simulink model "Obs_Avoi_with_sta_lin"  (R2023a)
settings: Solver=ode1  StartTime=0  StopTime=30  FixedStep=0.01  RelTol=1e-3
PostLoadFcn:
  | p=1:640; % pixels from left to right
  | 
  | Obtained_angles=(320-p).*(57/640)*pi./180;  % Kinect's horizontal FOV = 57 degrees
  | 
  | S=400; % S = Size of the 2D Map matrix... the highet S is the higher resolution we would end up with - %00 might be high for Embedded computing
values from neighbouring files (symbols this model uses):
  E = 0.3    [Main_Obst_Avoi_sta_lin.m]
  parameters = [R D omega Ts db  E b]    [Main_Obst_Avoi_sta_lin.m]
  Q0 = Qbd    [Main_Obst_Avoi_sta_lin.m]
  R = 0.035    [Main_Obst_Avoi_sta_lin.m]
  T = [R/2 R/2 ... (first row only)    [Main_Obst_Avoi_sta_lin.m]
  thetap = path.States(:,3)    [Main_Obst_Avoi_sta_lin.m]
  x = out.x.Data    [plots.m]
  X0 = p0    [Main_Obst_Avoi_sta_lin.m]
  xp = path.States(:,1)    [Main_Obst_Avoi_sta_lin.m]
  yp = path.States(:,2)    [Main_Obst_Avoi_sta_lin.m]
undefined symbols (not defined in the file or in its folder): gcbh, HIL, JPEG, qc_get_step_size, Video3D, video_display_show
libraries: quarc_library x29, simulink x3
(part 1 of 2)
settings Model: ExtModeTrigDuration=2  Creator=drmadill  LastModifiedBy=Ferna
settings SolverCC: AlgebraicLoopSolver=TrustRegion
settings DebuggingCC: UnderspecifiedInitializationDetection=Classic  MergeDetectMultiDrivingBlocksExec=none  UnconnectedInputMsg=warning  UnconnectedOutputMsg=warning  UnconnectedLineMsg=warning
settings ModelReferenceCC: EnableRefExpFcnMdlSchedulingChecks=on  PropagateSignalLabelsOutOfModel=off

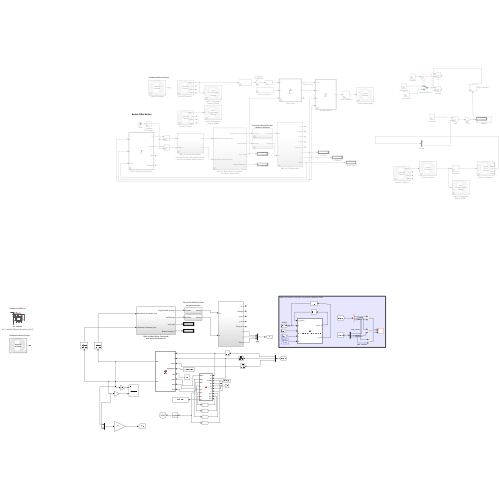
[thumbnail: Simulink's stored preview of the top-level diagram]
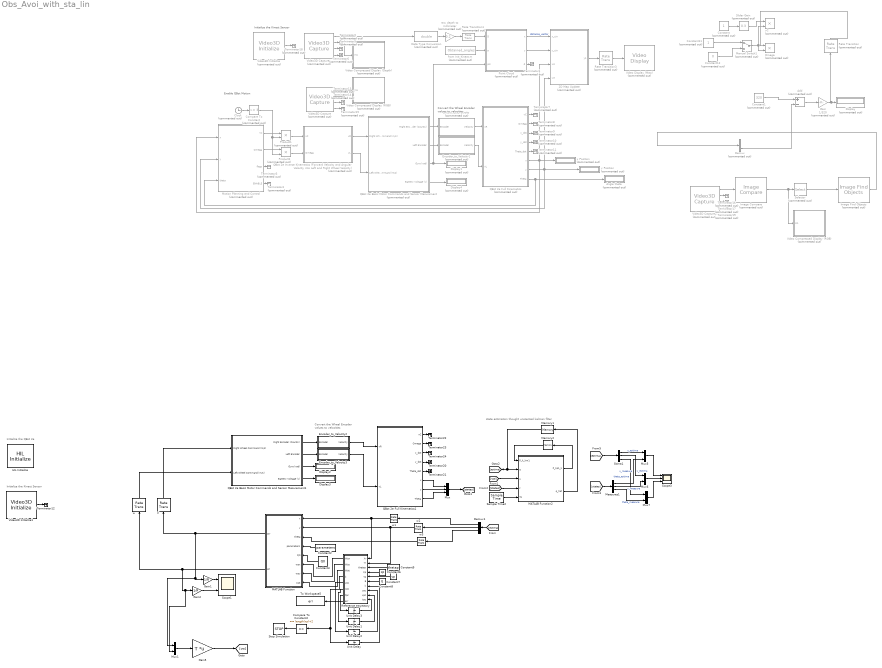
== system Obs_Avoi_with_sta_lin ==
  note: Enable QBot Motion
  note: Initialize the Kinect Sensor
  note: Initialize the QBot 2e
  note: Convert the Wheel Encoder
      | values to velocities
  note: Initialize the Kinect Sensor
  note: Convert the Wheel Encoder
      | values to velocities
  note: state estimation thought unscented kalman filter
  2D Map Update : MATLAB Function  Commented=on  TreatAsAtomicUnit=on  SystemSampleTime=qc_get_step_size
  Add : Sum  Commented=on  Inputs=+-
  Angle theta : Display  Commented=on
  Clock : Clock  Commented=on
  Compare To Constant : simulink/Logic and Bit Operations/Compare To Constant  Commented=on  relop=>=  const=3  OutDataTypeStr=boolean
  Compare To Constant2 : simulink/Logic and Bit Operations/Compare To Constant  relop===  const=length(xp)+2  OutDataTypeStr=boolean
  Constant : Constant  Commented=on
  Constant1 : Constant  Commented=on  Value=320
  Constant11 : Constant  Commented=on
  Constant12 : Constant  Commented=on  Value=0
  Constant2 : Constant  Value=parameters
  Constant3 : Constant  Value=Q0
  Constant6 : Constant  Value=xp
  Constant7 : Constant  Value=yp
  Constant8 : Constant  Value=E
  Constant9 : Constant  Value=thetap
  Data Type Conversion : DataTypeConversion  Commented=on  OutDataTypeStr=double  SaturateOnIntegerOverflow=off  RndMeth=Floor
  Demux : Demux  Commented=on  Outputs=2
  Demux1 : Demux  Outputs=3
  Display : Display  Commented=on
  Display1 : Display  Commented=on
  Display2 : Display
  Display3 : Display
  Display4 : Display  Commented=on
  Encoder_to_Velocity : Subsystem  Commented=on
  Encoder_to_Velocity1 : Subsystem  Commented=on
  Encoder_to_Velocity2 : Subsystem
  Encoder_to_Velocity3 : Subsystem
  Gain : Gain  Commented=on  Gain=1/320
  Gain1 : Gain  Gain=1/R
  Gain2 : Gain  Gain=1/R
  Gain5 : Gain  Gain=T  Multiplication=Matrix(K*u)
  HIL Initialize : quarc_library/Data Acquisition/Generic/Configuration/HIL Initialize  Priority=-99  object_name=HIL-1  board_type=qbot2e  board_number=0@tcpip://localhost:18910  board_options=pwm0_en=1;pwm0_pin=12;pwm1_en=1;pwm1_pin=13;  exclusive=off  active=on  hardware_clocks=[]  clock_modes=[]  initial_clock_frequencies=[]  set_clock_params_at_start=off  set_clock_params_at_switch_in=off  set_clock_frequencies_at_start=off  set_clock_frequencies_at_switch_in=off  analog_input_channels=[0:5]  analog_input_configurations=[]  analog_input_maximums=[16.5 3.3 3.3 3.3 3.3 3.3]  analog_input_minimums=[0 0 0 0 0 0]  set_analog_input_params_at_start=off  set_analog_input_params_at_switch_in=off  analog_output_channels=[]  analog_output_maximums=[]  analog_output_minimums=[]  initial_analog_outputs=[]  final_analog_outputs=[]  watchdog_analog_outputs=[]  set_analog_output_params_at_start=off  set_analog_output_params_at_switch_in=off  set_analog_outputs_at_start=off  set_analog_outputs_at_switch_in=off  set_analog_outputs_at_terminate=off  set_analog_outputs_at_switch_out=off  set_analog_outputs_on_watchdog=off  digital_input_channels=[28:58]  digital_output_channels=[28:31]  digital_output_configuration=[]  initial_digital_outputs=[0]  final_digital_outputs=[0]  watchdog_digital_outputs=[]  set_digital_output_params_at_start=off  set_digital_output_params_at_switch_in=off  set_digital_outputs_at_start=on  set_digital_outputs_at_switch_in=off  set_digital_outputs_at_terminate=on  set_digital_outputs_at_switch_out=off  set_digital_outputs_on_watchdog=off  encoder_channels=[0:1]  quadrature=[4]  encoder_filter_frequency=[]  initial_encoder_counts=[0]  set_encoder_params_at_start=on  set_encoder_params_at_switch_in=off  set_encoder_counts_at_start=on  set_encoder_counts_at_switch_in=off  pwm_channels=[0:1]  pwm_modes=0  pwm_frequency=100e6 / 4095  pwm_configuration=[0]  pwm_alignment=[0]  pwm_polarity=[1]  pwm_leading_deadband=[]  pwm_trailing_deadband=[]  initial_pwm_outputs=[0]  final_pwm_outputs=[0]  watchdog_pwm_outputs=[]  set_pwm_params_at_start=on  set_pwm_params_at_switch_in=off  set_pwm_outputs_at_start=on  set_pwm_outputs_at_switch_in=off  set_pwm_outputs_at_terminate=on  set_pwm_outputs_at_switch_out=off  set_pwm_outputs_on_watchdog=off  other_output_channels=[2000:2001 14000 16000]  initial_other_outputs=[0 0 0 7]  final_other_outputs=[0 0 0 7]  watchdog_other_outputs=[]  set_other_outputs_at_start=on  set_other_outputs_at_switch_in=off  set_other_outputs_at_terminate=on  set_other_outputs_at_switch_out=off  set_other_outputs_on_watchdog=off
  Image Compare : quarc_library/Image Processing/Generic/Image Compare  Commented=on  output_type=Combined (one HxW output)  source=Internal dialog parameters  r_comparison=min <= pixel and pixel <= max  r_minimum=180  r_maximum=255  g_comparison=min <= pixel and pixel <= max  g_minimum=0  g_maximum=50  b_comparison=min <= pixel and pixel <= max  b_minimum=0  b_maximum=50
      settings: SourceProductName=QUARC Targets
  Image Find Objects : quarc_library/Image Processing/Generic/Image Find Objects  Commented=on  num_objects=1  connectivity=8 directions (N, NE, E, SE, S, SW, W, NW)  sort_order=Sort by number of pixels  min_pixels=10  max_pixels=intmax('uint32')  largest=on  exclude_at_edges=off  variable_size=off  use_complex=off
      settings: SourceProductName=QUARC Targets
  MATLAB Function : MATLAB Function  TreatAsAtomicUnit=on
  MATLAB Function2 : MATLAB Function  TreatAsAtomicUnit=on
  Manual Switch1 : ManualSwitch  Commented=on
  Measures1 : Demux  Outputs=3
  Memory1 : Memory  InitialCondition=X0
  Memory2 : Memory  InitialCondition=1e-6*eye(3)
  Motion Planning and Control : MATLAB Function  Commented=on  TreatAsAtomicUnit=on  SystemSampleTime=qc_get_step_size
  Mux : Mux  Inputs=3
  Mux{1,5..7} (4 alike) : Mux  Inputs=2
  Omega : Product  Commented=on  Inputs=**
  Point Cloud : MATLAB Function  Commented=on  TreatAsAtomicUnit=on
  Product1 : Product  Commented=on  RndMeth=Zero
  Product2 : Product  Commented=on  RndMeth=Zero
  QBot 2e Basic Motor Commands and Sensor Mesurement : Subsystem  Commented=on
  QBot 2e Basic Motor Commands and Sensor Mesurement1 : Subsystem
  QBot 2e Full Kinematics : Subsystem  Commented=on
  QBot 2e Full Kinematics1 : Subsystem
  QBot 2e Inverse Kinematics (Forward Velocity and Angular Velocity into Left and Right Wheel Velocity) : Subsystem  Commented=on
  Rate Transition : RateTransition  Commented=on
  Rate Transition1 : RateTransition  Commented=on
  Rate Transition3 : RateTransition  Commented=on
  Reference trayectory : MATLAB Function  TreatAsAtomicUnit=on
  Sample Time2 : quarc_library/Sources/Time/Sample Time  Priority=-99  sample_time=Ts
  Scope1 : Scope  NumInputPorts=2
  Scope3 : Scope  NumInputPorts=3
  Selector : Selector  Commented=on  NumberOfDimensions=2  InputPortWidth=3  IndexOptions=Index vector (dialog),Select all  Indices=[300:480],1  OutputSizes=1,1
  Slider Gain : simulink/Math Operations/Slider Gain  Commented=on  gain=0.3  low=-1  high=1
  Stima1 : Demux  Outputs=3
  Stop Simulation : Stop
  Terminator{1..11,13..19} (18 alike) : Terminator  Commented=on
  Terminator{12,20..24} (6 alike) : Terminator
  To Workspace5 : ToWorkspace  VariableName=err  SaveFormat=Timeseries  SampleTime=-1
  Unit Delay : UnitDelay  InitialCondition=1  SampleTime=0.15  HasFrameUpgradeWarning=on
  Unit Delay1 : UnitDelay  InitialCondition=xp(1)  SampleTime=-1  HasFrameUpgradeWarning=on
  Unit Delay2 : UnitDelay  InitialCondition=yp(1)  SampleTime=-1  HasFrameUpgradeWarning=on
  Unit Delay3 : UnitDelay  InitialCondition=thetap(1)  SampleTime=-1  HasFrameUpgradeWarning=on
  V : RateTransition
  Video Compressed Display (Depth) : Subsystem  Commented=on  LoadFcn=set_param(gcbh, 'UserData', gcb);  StartFcn=video_display_show([gcb, '/Video Display'], 'add', gcb);  mask(Video Compressed Display){algorithm=JPEG, quality=50, sample_time=-1, use_hardware=on}
      mask prompts: algorithm "Compression algorithm:"; quality "Compression quality (0-100):"; sample_time "Sample time (seconds):"; use_hardware "Use hardware acceleration for video display"
      mask help: Displays a video stream on the host, using compression to minimize bandwidth.
      mask init:
      | qc_set_display('Video\nCompressed\nDisplay');
      settings: UndoDeleteFcn=set_param(gcbh, 'UserData', gcb);  OpenFcn=video_display_show([gcb, '/Video Display'], 'show', gcb);  PreDeleteFcn=video_display_show([gcb, '/Video Display'], 'delete');
      settings: CopyFcn=|
      | set_param(gcbh, 'UserData', gcb);
      | set_param(gcbh, 'LinkStatus', 'none');
      settings: NameChangeFcn=|
      | video_display_show([get_param(gcbh, 'UserData'), '/Video Display'], 'rename', [gcb, '/Video Display']);
      | video_display_show([gcb, '/Video Display'], 'add', gcb);
      | set_param(gcbh, 'UserData', gcb);
      mask Help: web(qc_get_block_help_path(gcb));
      mask TypeOptions algorithm: Image Compress/algorithm
      mask TypeOptions quality: Image Compress/quality
      mask TypeOptions sample_time: Video Display/sample_time
      mask TypeOptions use_hardware: Video Display/use_hardware
      mask Display:
      | patch([0.98591 0.98591 0.62618 0.59072 0.56147   0.536   0.536  0.5441 0.56912 0.59207 0.60881 0.62276 0.63527 0.64364  0.6485  0.6485 0.64706 0.64499 0.63662 0.62411 0.61232 0.59837 0.58307 0.56147   0.536   0.536  0.5441  0.5747 0.60953 0.63662 0.67001  0.7034 0.72851 0.75425 0.77927 0.80294 0.82454 0.84119 0.85865 0.87395 0.88574 0.89339  0.8969 0.89969 0.89969 0.89267  0.8816 0.87044 0.85649  0.8384 0.81824 0.80294 0.78764 0.77513 0.76676 0.75776 0.76397 0.77513 0.79178 0.80987 0.82796 0.84326 0.86207 0.98528],[0.18689 0.05522 0.05522 0.05171 0.05171    0.05 0.18338 0.18338 0.19148 0.20435 0.22298 0.24863 0.28589 0.33125 0.38138 0.55139 0.59801 0.63761 0.68189 0.72149 0.74939 0.76694 0.77855 0.79367 0.79952 0.92768 0.92768 0.92768 0.92417 0.92066 0.91364  0.9032 0.89384 0.88106 0.86594 0.85073 0.82634 0.80537 0.77855 0.74363 0.70403 0.65858 0.61079 0.59099 0.41513 0.37202 0.31847 0.29048 0.25556 0.23342  0.2102 0.19382 0.18221 0.17285 0.16943 0.16124  0.1589 0.16241 0.16709 0.17168  0.1787 0.18221 0.18689 0.18689],[0.9,0.90,0.91])
      | patch([0.536 0.52601 0.46823 0.44528 0.41603 0.39101 0.35555 0.33116 0.31451 0.29291  0.2804 0.26717 0.25322 0.23999 0.22406 0.20732 0.19337 0.17528 0.15935 0.14396 0.13217 0.11759 0.10922 0.10085 0.09671 0.09392 0.09041 0.08906 0.08906 0.09464  0.0995 0.10778 0.11894 0.13145 0.14675 0.16349 0.17672 0.19409 0.20732 0.22406 0.23999 0.26159 0.27833 0.29849 0.31793 0.33602 0.35411 0.37085 0.39245 0.41603   0.536   0.536 0.53159 0.46409   0.446 0.42026 0.39587 0.37571 0.36113 0.34925 0.34088 0.33809 0.33809 0.34088 0.34583 0.35627 0.36392 0.38129 0.39587 0.41117 0.42719 0.44672  0.4676 0.48353 0.48353 0.52394   0.536],[0.05 0.04829 0.04712 0.04712 0.04829 0.05063 0.05405 0.05873 0.06107 0.06692 0.07043 0.07619 0.08087 0.08672 0.09482 0.10652 0.11696 0.13325  0.1508 0.17168 0.19499 0.22415 0.25439 0.28472 0.31379 0.35456 0.38489 0.41513 0.58055 0.63878 0.68774 0.72149 0.75641 0.78089 0.80537 0.82859 0.84029 0.85658 0.86594 0.87404  0.8834 0.89267 0.90086 0.90788 0.91247 0.91832 0.92066   0.923 0.92651 0.92768 0.92768 0.79952 0.79952 0.79952 0.79718 0.78899 0.77153 0.75056 0.72149 0.68072 0.62249  0.5549 0.41396 0.37085 0.33242 0.28121 0.25205 0.22181 0.20552 0.19499 0.18572 0.18221 0.17753 0.17636 0.17753  0.1787  0.1787],[0.9,0.90,0.91])
      | disp('Video\nCompressed\nDisplay');
  Video Compressed Display (RGB) : Subsystem  Commented=on  LoadFcn=set_param(gcbh, 'UserData', gcb);  StartFcn=video_display_show([gcb, '/Video Display'], 'add', gcb);  mask(Video Compressed Display){algorithm=JPEG, quality=50, sample_time=-1, use_hardware=on}
      mask prompts: algorithm "Compression algorithm:"; quality "Compression quality (0-100):"; sample_time "Sample time (seconds):"; use_hardware "Use hardware acceleration for video display"
      mask help: Displays a video stream on the host, using compression to minimize bandwidth.
      mask init:
      | qc_set_display('Video\nCompressed\nDisplay');
      settings: UndoDeleteFcn=set_param(gcbh, 'UserData', gcb);  OpenFcn=video_display_show([gcb, '/Video Display'], 'show', gcb);  PreDeleteFcn=video_display_show([gcb, '/Video Display'], 'delete');
      settings: CopyFcn=|
      | set_param(gcbh, 'UserData', gcb);
      | set_param(gcbh, 'LinkStatus', 'none');
      settings: NameChangeFcn=|
      | video_display_show([get_param(gcbh, 'UserData'), '/Video Display'], 'rename', [gcb, '/Video Display']);
      | video_display_show([gcb, '/Video Display'], 'add', gcb);
      | set_param(gcbh, 'UserData', gcb);
      mask Help: web(qc_get_block_help_path(gcb));
      mask TypeOptions algorithm: Image Compress/algorithm
      mask TypeOptions quality: Image Compress/quality
      mask TypeOptions sample_time: Video Display/sample_time
      mask TypeOptions use_hardware: Video Display/use_hardware
      mask Display:
      | patch([0.98591 0.98591 0.62618 0.59072 0.56147   0.536   0.536  0.5441 0.56912 0.59207 0.60881 0.62276 0.63527 0.64364  0.6485  0.6485 0.64706 0.64499 0.63662 0.62411 0.61232 0.59837 0.58307 0.56147   0.536   0.536  0.5441  0.5747 0.60953 0.63662 0.67001  0.7034 0.72851 0.75425 0.77927 0.80294 0.82454 0.84119 0.85865 0.87395 0.88574 0.89339  0.8969 0.89969 0.89969 0.89267  0.8816 0.87044 0.85649  0.8384 0.81824 0.80294 0.78764 0.77513 0.76676 0.75776 0.76397 0.77513 0.79178 0.80987 0.82796 0.84326 0.86207 0.98528],[0.18689 0.05522 0.05522 0.05171 0.05171    0.05 0.18338 0.18338 0.19148 0.20435 0.22298 0.24863 0.28589 0.33125 0.38138 0.55139 0.59801 0.63761 0.68189 0.72149 0.74939 0.76694 0.77855 0.79367 0.79952 0.92768 0.92768 0.92768 0.92417 0.92066 0.91364  0.9032 0.89384 0.88106 0.86594 0.85073 0.82634 0.80537 0.77855 0.74363 0.70403 0.65858 0.61079 0.59099 0.41513 0.37202 0.31847 0.29048 0.25556 0.23342  0.2102 0.19382 0.18221 0.17285 0.16943 0.16124  0.1589 0.16241 0.16709 0.17168  0.1787 0.18221 0.18689 0.18689],[0.9,0.90,0.91])
      | patch([0.536 0.52601 0.46823 0.44528 0.41603 0.39101 0.35555 0.33116 0.31451 0.29291  0.2804 0.26717 0.25322 0.23999 0.22406 0.20732 0.19337 0.17528 0.15935 0.14396 0.13217 0.11759 0.10922 0.10085 0.09671 0.09392 0.09041 0.08906 0.08906 0.09464  0.0995 0.10778 0.11894 0.13145 0.14675 0.16349 0.17672 0.19409 0.20732 0.22406 0.23999 0.26159 0.27833 0.29849 0.31793 0.33602 0.35411 0.37085 0.39245 0.41603   0.536   0.536 0.53159 0.46409   0.446 0.42026 0.39587 0.37571 0.36113 0.34925 0.34088 0.33809 0.33809 0.34088 0.34583 0.35627 0.36392 0.38129 0.39587 0.41117 0.42719 0.44672  0.4676 0.48353 0.48353 0.52394   0.536],[0.05 0.04829 0.04712 0.04712 0.04829 0.05063 0.05405 0.05873 0.06107 0.06692 0.07043 0.07619 0.08087 0.08672 0.09482 0.10652 0.11696 0.13325  0.1508 0.17168 0.19499 0.22415 0.25439 0.28472 0.31379 0.35456 0.38489 0.41513 0.58055 0.63878 0.68774 0.72149 0.75641 0.78089 0.80537 0.82859 0.84029 0.85658 0.86594 0.87404  0.8834 0.89267 0.90086 0.90788 0.91247 0.91832 0.92066   0.923 0.92651 0.92768 0.92768 0.79952 0.79952 0.79952 0.79718 0.78899 0.77153 0.75056 0.72149 0.68072 0.62249  0.5549 0.41396 0.37085 0.33242 0.28121 0.25205 0.22181 0.20552 0.19499 0.18572 0.18221 0.17753 0.17636 0.17753  0.1787  0.1787],[0.9,0.90,0.91])
      | disp('Video\nCompressed\nDisplay');
  "Video Compressed Display (RGB) " : Subsystem  Commented=on  LoadFcn=set_param(gcbh, 'UserData', gcb);  StartFcn=video_display_show([gcb, '/Video Display'], 'add', gcb);  mask(Video Compressed Display){algorithm=JPEG, quality=50, sample_time=-1, use_hardware=on}
      mask prompts: algorithm "Compression algorithm:"; quality "Compression quality (0-100):"; sample_time "Sample time (seconds):"; use_hardware "Use hardware acceleration for video display"
      mask help: Displays a video stream on the host, using compression to minimize bandwidth.
      mask init:
      | qc_set_display('Video\nCompressed\nDisplay');
      settings: UndoDeleteFcn=set_param(gcbh, 'UserData', gcb);  OpenFcn=video_display_show([gcb, '/Video Display'], 'show', gcb);  PreDeleteFcn=video_display_show([gcb, '/Video Display'], 'delete');
      settings: CopyFcn=|
      | set_param(gcbh, 'UserData', gcb);
      | set_param(gcbh, 'LinkStatus', 'none');
      settings: NameChangeFcn=|
      | video_display_show([get_param(gcbh, 'UserData'), '/Video Display'], 'rename', [gcb, '/Video Display']);
      | video_display_show([gcb, '/Video Display'], 'add', gcb);
      | set_param(gcbh, 'UserData', gcb);
      mask Help: web(qc_get_block_help_path(gcb));
      mask TypeOptions algorithm: Image Compress/algorithm
      mask TypeOptions quality: Image Compress/quality
      mask TypeOptions sample_time: Video Display/sample_time
      mask TypeOptions use_hardware: Video Display/use_hardware
      mask Display:
      | patch([0.98591 0.98591 0.62618 0.59072 0.56147   0.536   0.536  0.5441 0.56912 0.59207 0.60881 0.62276 0.63527 0.64364  0.6485  0.6485 0.64706 0.64499 0.63662 0.62411 0.61232 0.59837 0.58307 0.56147   0.536   0.536  0.5441  0.5747 0.60953 0.63662 0.67001  0.7034 0.72851 0.75425 0.77927 0.80294 0.82454 0.84119 0.85865 0.87395 0.88574 0.89339  0.8969 0.89969 0.89969 0.89267  0.8816 0.87044 0.85649  0.8384 0.81824 0.80294 0.78764 0.77513 0.76676 0.75776 0.76397 0.77513 0.79178 0.80987 0.82796 0.84326 0.86207 0.98528],[0.18689 0.05522 0.05522 0.05171 0.05171    0.05 0.18338 0.18338 0.19148 0.20435 0.22298 0.24863 0.28589 0.33125 0.38138 0.55139 0.59801 0.63761 0.68189 0.72149 0.74939 0.76694 0.77855 0.79367 0.79952 0.92768 0.92768 0.92768 0.92417 0.92066 0.91364  0.9032 0.89384 0.88106 0.86594 0.85073 0.82634 0.80537 0.77855 0.74363 0.70403 0.65858 0.61079 0.59099 0.41513 0.37202 0.31847 0.29048 0.25556 0.23342  0.2102 0.19382 0.18221 0.17285 0.16943 0.16124  0.1589 0.16241 0.16709 0.17168  0.1787 0.18221 0.18689 0.18689],[0.9,0.90,0.91])
      | patch([0.536 0.52601 0.46823 0.44528 0.41603 0.39101 0.35555 0.33116 0.31451 0.29291  0.2804 0.26717 0.25322 0.23999 0.22406 0.20732 0.19337 0.17528 0.15935 0.14396 0.13217 0.11759 0.10922 0.10085 0.09671 0.09392 0.09041 0.08906 0.08906 0.09464  0.0995 0.10778 0.11894 0.13145 0.14675 0.16349 0.17672 0.19409 0.20732 0.22406 0.23999 0.26159 0.27833 0.29849 0.31793 0.33602 0.35411 0.37085 0.39245 0.41603   0.536   0.536 0.53159 0.46409   0.446 0.42026 0.39587 0.37571 0.36113 0.34925 0.34088 0.33809 0.33809 0.34088 0.34583 0.35627 0.36392 0.38129 0.39587 0.41117 0.42719 0.44672  0.4676 0.48353 0.48353 0.52394   0.536],[0.05 0.04829 0.04712 0.04712 0.04829 0.05063 0.05405 0.05873 0.06107 0.06692 0.07043 0.07619 0.08087 0.08672 0.09482 0.10652 0.11696 0.13325  0.1508 0.17168 0.19499 0.22415 0.25439 0.28472 0.31379 0.35456 0.38489 0.41513 0.58055 0.63878 0.68774 0.72149 0.75641 0.78089 0.80537 0.82859 0.84029 0.85658 0.86594 0.87404  0.8834 0.89267 0.90086 0.90788 0.91247 0.91832 0.92066   0.923 0.92651 0.92768 0.92768 0.79952 0.79952 0.79952 0.79718 0.78899 0.77153 0.75056 0.72149 0.68072 0.62249  0.5549 0.41396 0.37085 0.33242 0.28121 0.25205 0.22181 0.20552 0.19499 0.18572 0.18221 0.17753 0.17636 0.17753  0.1787  0.1787],[0.9,0.90,0.91])
      | disp('Video\nCompressed\nDisplay');
  Video Display (Map) : quarc_library/Multimedia/Video Display  Tag=Obs_Avoi_with_sta_lin/Video Display (Map)  Commented=on  sample_time=-1  use_hardware=on
  Video3D Capture : quarc_library/Multimedia/Video3D Capture  Commented=on  object_name=Video3D-1  stream_type=RGB  stream_index=0  resolution=640 x 480  width=640  height=480  output_format=MATLAB RGB (HxWx3)  data_type=uint8  sample_time=qc_get_step_size * ceil(0.033 / qc_get_step_size)  camera_intrinsics=off  depth_scale=off  brightness_override=off  brightness=50.0  contrast_override=off  contrast=50.0  hue_override=off  hue=50.0  saturation_override=off  saturation=50.0  sharpness_override=off  sharpness=50.0  gamma_override=off  gamma=50.0  gain_override=off  gain=50.0  backlightcompensation_override=off  backlightcompensation=50.0  whitebalance_override=Automatic white balance  whitebalance=50.0  exposure_override=Automatic exposure  exposure=30.0  emitter=Enable laser emitter  preset=Do not set camera presets
  Video3D Capture1 : quarc_library/Multimedia/Video3D Capture  Commented=on  object_name=Video3D-1  stream_type=Depth  stream_index=0  resolution=640 x 480  width=640  height=480  output_format=MATLAB greyscale (HxW)  data_type=uint16  sample_time=qc_get_step_size * ceil(0.033 / qc_get_step_size)  camera_intrinsics=off  depth_scale=off  brightness_override=off  brightness=50.0  contrast_override=off  contrast=50.0  hue_override=off  hue=50.0  saturation_override=off  saturation=50.0  sharpness_override=off  sharpness=50.0  gamma_override=off  gamma=50.0  gain_override=off  gain=50.0  backlightcompensation_override=off  backlightcompensation=50.0  whitebalance_override=Automatic white balance  whitebalance=50.0  exposure_override=Automatic exposure  exposure=30.0  emitter=Enable laser emitter  preset=Do not set camera presets
  Video3D Capture2 : quarc_library/Multimedia/Video3D Capture  Commented=on  object_name=Video3D-1  stream_type=RGB  stream_index=0  resolution=640 x 480  width=640  height=480  output_format=MATLAB RGB (HxWx3)  data_type=uint8  sample_time=qc_get_step_size * ceil(0.033 / qc_get_step_size)  camera_intrinsics=off  depth_scale=off  brightness_override=off  brightness=50.0  contrast_override=off  contrast=50.0  hue_override=off  hue=50.0  saturation_override=off  saturation=50.0  sharpness_override=off  sharpness=50.0  gamma_override=off  gamma=50.0  gain_override=off  gain=50.0  backlightcompensation_override=off  backlightcompensation=50.0  whitebalance_override=Automatic white balance  whitebalance=50.0  exposure_override=Automatic exposure  exposure=30.0  emitter=Enable laser emitter  preset=Do not set camera presets
  Video3D Initialize : quarc_library/Multimedia/Video3D Initialize  Commented=on  object_name=Video3D-1  source=Device  identifier=0@tcpip://localhost:18911  file=sample.bag  sample_time=qc_get_step_size * ceil(0.033 / qc_get_step_size)  active=on
  Video3D Initialize1 : quarc_library/Multimedia/Video3D Initialize  object_name=Video3D-1  source=Device  identifier=0@tcpip://localhost:18911  file=sample.bag  sample_time=qc_get_step_size * ceil(0.033 / qc_get_step_size)  active=on
  from Init_Kinect.m : Constant  Commented=on  Value=Obtained_angles
  raw depth to millimeter : Gain  Commented=on  Gain=0.2  OutDataTypeStr=single
  vC : Product  Commented=on  Inputs=**
  w : RateTransition
  w1 : RateTransition  OutPortSampleTime=Ts
  w2 : RateTransition  OutPortSampleTime=Ts
  w3 : RateTransition  OutPortSampleTime=Ts
  x Position : Display  Commented=on
  y Position : Display  Commented=on
  wires:
  QBot 2e Basic Motor Commands and Sensor Mesurement/1(Right Encoder (Counts)) -> Encoder_to_Velocity/1(Encoder)
  QBot 2e Full Kinematics/8(Theta) -> Motion Planning and Control/3(theta), Angle theta/1
  QBot 2e Full Kinematics/6(x) -> Motion Planning and Control/1(x), x Position/1, 2D Map Update/3(xin)
  from Init_Kinect.m/1 -> Point Cloud/2(a)
  Point Cloud/1(x) -> 2D Map Update/1(x_cin)  "distance_vector"
  Point Cloud/2(y) -> 2D Map Update/2(y_cin)
  2D Map Update/1(y1) -> Rate Transition3/1
  Video3D Capture1/1 -> Video Compressed Display (Depth)/1(In1), Data Type Conversion/1
  QBot 2e Basic Motor Commands and Sensor Mesurement/3(Gyro (rad)) -> Point Cloud/3(psi), Display1/1
  QBot 2e Basic Motor Commands and Sensor Mesurement/4(Battery Voltage (v)) -> Display4/1
  Encoder_to_Velocity/1(Velocity) -> QBot 2e Full Kinematics/1(vR)
  QBot 2e Inverse Kinematics (Forward Velocity and Angular Velocity into Left and Right Wheel Velocity)/2(vL) -> QBot 2e Basic Motor Commands and Sensor Mesurement/2(Left Wheel Command (m/s))
  QBot 2e Basic Motor Commands and Sensor Mesurement/2(Left Encoder) -> Encoder_to_Velocity1/1(Encoder)
  Encoder_to_Velocity1/1(Velocity) -> QBot 2e Full Kinematics/2(vL)
  Motion Planning and Control/1(Vc) -> Product1/1
  Product1/1 -> QBot 2e Inverse Kinematics (Forward Velocity and Angular Velocity into Left and Right Wheel Velocity)/1(vC)
  Motion Planning and Control/2(Omega) -> Product2/1
  Product2/1 -> QBot 2e Inverse Kinematics (Forward Velocity and Angular Velocity into Left and Right Wheel Velocity)/2(Omega)
  Compare To Constant/1 -> Product2/2, Product1/2
  QBot 2e Inverse Kinematics (Forward Velocity and Angular Velocity into Left and Right Wheel Velocity)/1(vR) -> QBot 2e Basic Motor Commands and Sensor Mesurement/1(Right Wheel Command (m/s))
  Motion Planning and Control/3(flags) -> Terminator3/1
  Motion Planning and Control/4(ENABLE) -> Terminator4/1
  QBot 2e Full Kinematics/7(y) -> y Position/1, 2D Map Update/4(yin), Motion Planning and Control/2(y)
  QBot 2e Full Kinematics/1(vC) -> Terminator7/1
  QBot 2e Full Kinematics/2(Omega) -> Terminator8/1
  QBot 2e Full Kinematics/3(x_dot) -> Terminator9/1
  QBot 2e Full Kinematics/4(y_dot) -> Terminator10/1
  QBot 2e Full Kinematics/5(Theta_dot) -> Terminator11/1
  Rate Transition3/1 -> Video Display (Map)/1
  Video3D Capture/1 -> Video Compressed Display (RGB)/1(In1)
  Point Cloud/3(d) -> Terminator1/1
  Video3D Capture/2 -> Terminator13/1
  Video3D Capture/4 -> Terminator15/1
  Video3D Capture/3 -> Terminator14/1
  Video3D Initialize/1 -> Terminator18/1
  Video3D Capture1/2 -> Terminator2/1
  Video3D Capture1/3 -> Terminator5/1
  Video3D Capture1/4 -> Terminator6/1
  Rate Transition1/1 -> Point Cloud/1(D)
  raw depth to millimeter/1 -> Rate Transition1/1
  Data Type Conversion/1 -> raw depth to millimeter/1
  Clock/1 -> Compare To Constant/1
  Constant/1 -> Slider Gain/1
  Video3D Initialize1/1 -> Terminator12/1
  Video3D Capture2/4 -> Terminator19/1
  Video3D Capture2/2 -> Terminator16/1
  Video3D Capture2/1 -> Image Compare/1
  Video3D Capture2/3 -> Terminator17/1
  Image Compare/1 -> "Video Compressed Display (RGB) "/1(In1), Selector/1
  Selector/1 -> Image Find Objects/1
  Image Find Objects/3 -> Demux/1
  Demux/2 -> Add/2
  Constant1/1 -> Add/1
  Add/1 -> Gain/1
  Gain/1 -> Rate Transition/1, Display/1
  QBot 2e Basic Motor Commands and Sensor Mesurement1/1(Right Encoder (Counts)) -> Encoder_to_Velocity2/1(Encoder)
  QBot 2e Basic Motor Commands and Sensor Mesurement1/2(Left Encoder) -> Encoder_to_Velocity3/1(Encoder)
  QBot 2e Basic Motor Commands and Sensor Mesurement1/4(Battery Voltage (v)) -> Display3/1
  QBot 2e Basic Motor Commands and Sensor Mesurement1/3(Gyro (rad)) -> Display2/1
  QBot 2e Full Kinematics1/4(y_dot) -> Terminator20/1
  QBot 2e Full Kinematics1/3(x_dot) -> Terminator24/1
  Encoder_to_Velocity2/1(Velocity) -> QBot 2e Full Kinematics1/1(vR)
  QBot 2e Full Kinematics1/5(Theta_dot) -> Terminator21/1
  QBot 2e Full Kinematics1/2(Omega) -> Terminator23/1
  QBot 2e Full Kinematics1/1(vC) -> Terminator22/1
  Encoder_to_Velocity3/1(Velocity) -> QBot 2e Full Kinematics1/2(vL)
  QBot 2e Full Kinematics1/6(x) -> Mux/1
  QBot 2e Full Kinematics1/8(Theta) -> Mux/3
  w1/1 -> Reference trayectory/1(Xr), MATLAB Function/1(x)
  w3/1 -> MATLAB Function/3(theta)
  MATLAB Function/1(Wr) -> V/1, Mux1/1, Gain1/1
  Reference trayectory/1(Wpx) -> MATLAB Function/6(wpx)
  Reference trayectory/2(Wpy) -> MATLAB Function/7(wpy)
  Constant2/1 -> MATLAB Function/4(parameters)
  Constant3/1 -> MATLAB Function/5(Q0)
  Slider Gain/1 -> vC/1
  Constant12/1 -> Manual Switch1/2
  Constant11/1 -> Manual Switch1/1
  Manual Switch1/1 -> Omega/2, vC/2
  Rate Transition/1 -> Omega/1
  w2/1 -> Reference trayectory/2(Yr), MATLAB Function/2(y)
  QBot 2e Full Kinematics1/7(y) -> Mux/2
  MATLAB Function/2(Wl) -> w/1, Mux1/2, Gain2/1
  w/1 -> QBot 2e Basic Motor Commands and Sensor Mesurement1/2(Left Wheel Command (m/s))
  V/1 -> QBot 2e Basic Motor Commands and Sensor Mesurement1/1(Right Wheel Command (m/s))
  Gain1/1 -> Scope1/1
  Gain2/1 -> Scope1/2
  Constant6/1 -> Reference trayectory/4(Xp)
  Constant7/1 -> Reference trayectory/5(Yp)
  Constant8/1 -> Reference trayectory/6(E)
  Reference trayectory/4(k) -> Compare To Constant2/1, Unit Delay/1
  Unit Delay/1 -> Reference trayectory/7("k ")
  Unit Delay1/1 -> Reference trayectory/9("xpc ")
  Unit Delay2/1 -> Reference trayectory/8("ypc ")
  Reference trayectory/6(xpc) -> Unit Delay1/1
  Reference trayectory/5(ypc) -> Unit Delay2/1
  Constant9/1 -> Reference trayectory/3(thetap)
  Reference trayectory/7(tpc) -> Unit Delay3/1
  Unit Delay3/1 -> Reference trayectory/10("tpc ")
  Reference trayectory/3(Wpt) -> MATLAB Function/8(wpt)
  Compare To Constant2/1 -> Stop Simulation/1
  Demux1/1 -> w1/1
  Demux1/2 -> w2/1
  Demux1/3 -> w3/1
  Mux1/1 -> Gain5/1
  Reference trayectory/8(err) -> To Workspace5/1
  Stima1/2 -> Mux6/1  "y_estima"
  Measures1/3 -> Mux7/2  "theta_measure"
  Mux7/1 -> Scope3/3
  [states] -> Measures1/1
  Stima1/3 -> Mux7/1  "theta_estima"
  MATLAB Function2/1(P_kp1_k) -> Memory2/1
  Measures1/1 -> Mux5/2  "x_measure"
  Mux6/1 -> Scope3/2
  [estima] -> Stima1/1
  [vw] -> MATLAB Function2/3(u)
  [states] -> MATLAB Function2/4(y)
  Memory2/1 -> MATLAB Function2/1(P_k_km1)
  Sample Time2/1 -> MATLAB Function2/5(Ts)
  MATLAB Function2/2(q_hat) -> Memory1/1
  Stima1/1 -> Mux5/1  "x_estima"
  Mux5/1 -> Scope3/1
  Memory1/1 -> MATLAB Function2/2(q), [estima]
  Measures1/2 -> Mux6/2  "y_measure"
  Mux/1 -> [states]
  [estima] -> Demux1/1
  Gain5/1 -> [vw]

== system Obs_Avoi_with_sta_lin/Encoder_to_Velocity ==
  Encoder : Inport
  Encoder to Distance : Subsystem
  Second-Order Low-Pass Filter2 : quarc_library/Continuous/Second-Order Low-Pass Filter  params_source=Internal (dialog parameters)  input_width=10  input_zeta=1  input_init=0
  Terminator1 : Terminator
  Velocity : Outport  VectorParamsAs1DForOutWhenUnconnected=off
  wires:
  Second-Order Low-Pass Filter2/1 -> Terminator1/1
  Encoder to Distance/1(Wheel Distance (m)) -> Second-Order Low-Pass Filter2/1
  Encoder/1 -> Encoder to Distance/1(Encoder Counts)
  Second-Order Low-Pass Filter2/2 -> Velocity/1

== system Obs_Avoi_with_sta_lin/Encoder_to_Velocity1 ==
  Encoder : Inport
  Encoder to Distance : Subsystem
  Second-Order Low-Pass Filter2 : quarc_library/Continuous/Second-Order Low-Pass Filter  params_source=Internal (dialog parameters)  input_width=10  input_zeta=1  input_init=0
  Terminator1 : Terminator
  Velocity : Outport  VectorParamsAs1DForOutWhenUnconnected=off
  wires:
  Second-Order Low-Pass Filter2/2 -> Velocity/1
  Encoder/1 -> Encoder to Distance/1(Encoder Counts)
  Encoder to Distance/1(Wheel Distance (m)) -> Second-Order Low-Pass Filter2/1
  Second-Order Low-Pass Filter2/1 -> Terminator1/1

== system Obs_Avoi_with_sta_lin/Encoder_to_Velocity2 ==
  Encoder : Inport
  Encoder to Distance : Subsystem
  Second-Order Low-Pass Filter2 : quarc_library/Continuous/Second-Order Low-Pass Filter  params_source=Internal (dialog parameters)  input_width=10  input_zeta=1  input_init=0
  Terminator1 : Terminator
  Velocity : Outport  VectorParamsAs1DForOutWhenUnconnected=off
  wires:
  Second-Order Low-Pass Filter2/1 -> Terminator1/1
  Encoder to Distance/1(Wheel Distance (m)) -> Second-Order Low-Pass Filter2/1
  Encoder/1 -> Encoder to Distance/1(Encoder Counts)
  Second-Order Low-Pass Filter2/2 -> Velocity/1

== system Obs_Avoi_with_sta_lin/Encoder_to_Velocity3 ==
  Encoder : Inport
  Encoder to Distance : Subsystem
  Second-Order Low-Pass Filter2 : quarc_library/Continuous/Second-Order Low-Pass Filter  params_source=Internal (dialog parameters)  input_width=10  input_zeta=1  input_init=0
  Terminator1 : Terminator
  Velocity : Outport  VectorParamsAs1DForOutWhenUnconnected=off
  wires:
  Second-Order Low-Pass Filter2/2 -> Velocity/1
  Encoder/1 -> Encoder to Distance/1(Encoder Counts)
  Encoder to Distance/1(Wheel Distance (m)) -> Second-Order Low-Pass Filter2/1
  Second-Order Low-Pass Filter2/1 -> Terminator1/1

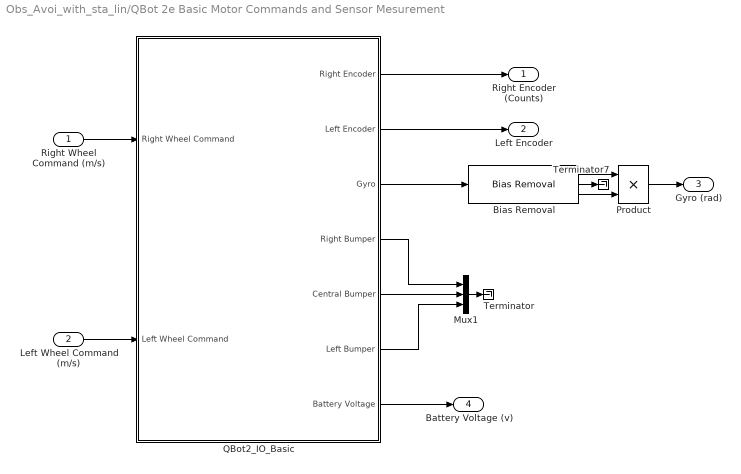
== system Obs_Avoi_with_sta_lin/QBot 2e Basic Motor Commands and Sensor Mesurement ==
  Right Wheel Command (m/s) : Inport
  Left Wheel Command (m/s) : Inport  Port=2
  Bias Removal : quarc_library/Discrete/Bias Removal  start_time=3  end_time=4  switch_id=0  sample_time=qc_get_step_size
      settings: SourceProductName=QUARC Targets
  Mux1 : Mux  Inputs=3
  Product : Product  RndMeth=Zero
  QBot2_IO_Basic : Subsystem
  Terminator : Terminator
  Terminator7 : Terminator
  Right Encoder (Counts) : Outport  VectorParamsAs1DForOutWhenUnconnected=off
  Left Encoder : Outport  Port=2  VectorParamsAs1DForOutWhenUnconnected=off
  Gyro (rad) : Outport  Port=3  VectorParamsAs1DForOutWhenUnconnected=off
  Battery Voltage (v) : Outport  Port=4  VectorParamsAs1DForOutWhenUnconnected=off
  wires:
  QBot2_IO_Basic/4(Right Bumper) -> Mux1/1
  QBot2_IO_Basic/5(Central Bumper) -> Mux1/2
  QBot2_IO_Basic/6(Left Bumper) -> Mux1/3
  Right Wheel Command (m/s)/1 -> QBot2_IO_Basic/1(Right Wheel Command)
  Left Wheel Command (m/s)/1 -> QBot2_IO_Basic/2(Left Wheel Command)
  QBot2_IO_Basic/1(Right Encoder) -> Right Encoder (Counts)/1
  QBot2_IO_Basic/2(Left Encoder) -> Left Encoder/1
  QBot2_IO_Basic/7(Battery Voltage) -> Battery Voltage (v)/1
  Bias Removal/2 -> Terminator7/1
  Bias Removal/1 -> Product/1
  Bias Removal/3 -> Product/2
  Product/1 -> Gyro (rad)/1
  QBot2_IO_Basic/3(Gyro) -> Bias Removal/1
  Mux1/1 -> Terminator/1

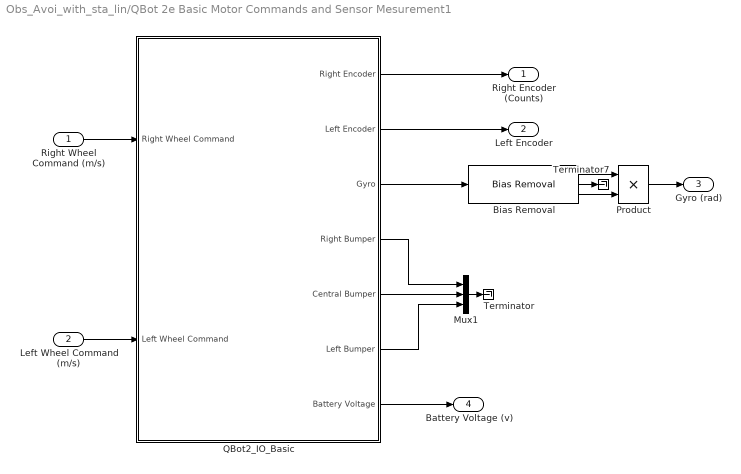
== system Obs_Avoi_with_sta_lin/QBot 2e Basic Motor Commands and Sensor Mesurement1 ==
  Right Wheel Command (m/s) : Inport
  Left Wheel Command (m/s) : Inport  Port=2
  Bias Removal : quarc_library/Discrete/Bias Removal  start_time=3  end_time=4  switch_id=0  sample_time=qc_get_step_size
      settings: SourceProductName=QUARC Targets
  Mux1 : Mux  Inputs=3
  Product : Product  RndMeth=Zero
  QBot2_IO_Basic : Subsystem
  Terminator : Terminator
  Terminator7 : Terminator
  Right Encoder (Counts) : Outport  VectorParamsAs1DForOutWhenUnconnected=off
  Left Encoder : Outport  Port=2  VectorParamsAs1DForOutWhenUnconnected=off
  Gyro (rad) : Outport  Port=3  VectorParamsAs1DForOutWhenUnconnected=off
  Battery Voltage (v) : Outport  Port=4  VectorParamsAs1DForOutWhenUnconnected=off
  wires:
  QBot2_IO_Basic/4(Right Bumper) -> Mux1/1
  QBot2_IO_Basic/5(Central Bumper) -> Mux1/2
  QBot2_IO_Basic/6(Left Bumper) -> Mux1/3
  Right Wheel Command (m/s)/1 -> QBot2_IO_Basic/1(Right Wheel Command)
  Left Wheel Command (m/s)/1 -> QBot2_IO_Basic/2(Left Wheel Command)
  QBot2_IO_Basic/1(Right Encoder) -> Right Encoder (Counts)/1
  QBot2_IO_Basic/2(Left Encoder) -> Left Encoder/1
  QBot2_IO_Basic/7(Battery Voltage) -> Battery Voltage (v)/1
  Bias Removal/2 -> Terminator7/1
  Bias Removal/1 -> Product/1
  Bias Removal/3 -> Product/2
  Product/1 -> Gyro (rad)/1
  QBot2_IO_Basic/3(Gyro) -> Bias Removal/1
  Mux1/1 -> Terminator/1

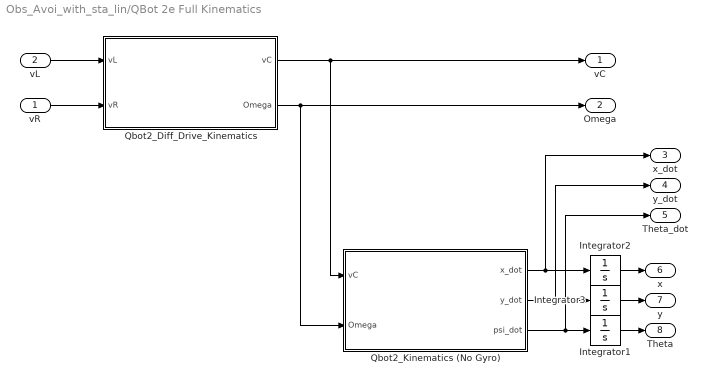
== system Obs_Avoi_with_sta_lin/QBot 2e Full Kinematics ==
  vR : Inport
  vL : Inport  Port=2
  Integrator1 : Integrator
  Integrator2 : Integrator
  Integrator3 : Integrator
  Qbot2_Diff_Drive_Kinematics : Subsystem
  Qbot2_Kinematics (No Gyro) : Subsystem
  vC : Outport  VectorParamsAs1DForOutWhenUnconnected=off
  Omega : Outport  Port=2  VectorParamsAs1DForOutWhenUnconnected=off
  x_dot : Outport  Port=3  VectorParamsAs1DForOutWhenUnconnected=off
  y_dot : Outport  Port=4  VectorParamsAs1DForOutWhenUnconnected=off
  Theta_dot : Outport  Port=5  VectorParamsAs1DForOutWhenUnconnected=off
  x : Outport  Port=6  VectorParamsAs1DForOutWhenUnconnected=off
  y : Outport  Port=7  VectorParamsAs1DForOutWhenUnconnected=off
  Theta : Outport  Port=8  VectorParamsAs1DForOutWhenUnconnected=off
  wires:
  Integrator1/1 -> Theta/1
  Qbot2_Kinematics (No Gyro)/3(psi_dot) -> Theta_dot/1, Integrator1/1
  Qbot2_Kinematics (No Gyro)/1(x_dot) -> x_dot/1, Integrator2/1
  Qbot2_Kinematics (No Gyro)/2(y_dot) -> y_dot/1, Integrator3/1
  Qbot2_Diff_Drive_Kinematics/1(vC) -> Qbot2_Kinematics (No Gyro)/1(vC), vC/1
  vL/1 -> Qbot2_Diff_Drive_Kinematics/1(vL)
  vR/1 -> Qbot2_Diff_Drive_Kinematics/2(vR)
  Integrator2/1 -> x/1
  Integrator3/1 -> y/1
  Qbot2_Diff_Drive_Kinematics/2(Omega) -> Qbot2_Kinematics (No Gyro)/2(Omega), Omega/1

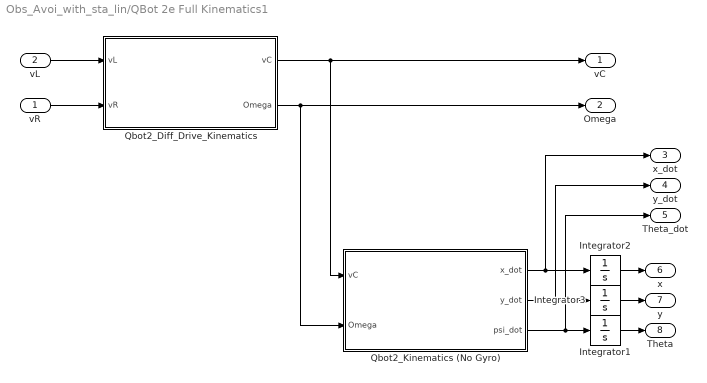
== system Obs_Avoi_with_sta_lin/QBot 2e Full Kinematics1 ==
  vR : Inport
  vL : Inport  Port=2
  Integrator1 : Integrator  InitialCondition=X0(3)
  Integrator2 : Integrator  InitialCondition=X0(1)
  Integrator3 : Integrator  InitialCondition=X0(2)
  Qbot2_Diff_Drive_Kinematics : Subsystem
  Qbot2_Kinematics (No Gyro) : Subsystem
  vC : Outport  VectorParamsAs1DForOutWhenUnconnected=off
  Omega : Outport  Port=2  VectorParamsAs1DForOutWhenUnconnected=off
  x_dot : Outport  Port=3  VectorParamsAs1DForOutWhenUnconnected=off
  y_dot : Outport  Port=4  VectorParamsAs1DForOutWhenUnconnected=off
  Theta_dot : Outport  Port=5  VectorParamsAs1DForOutWhenUnconnected=off
  x : Outport  Port=6  VectorParamsAs1DForOutWhenUnconnected=off
  y : Outport  Port=7  VectorParamsAs1DForOutWhenUnconnected=off
  Theta : Outport  Port=8  VectorParamsAs1DForOutWhenUnconnected=off
  wires:
  Integrator1/1 -> Theta/1
  Qbot2_Kinematics (No Gyro)/3(psi_dot) -> Theta_dot/1, Integrator1/1
  Qbot2_Kinematics (No Gyro)/1(x_dot) -> x_dot/1, Integrator2/1
  Qbot2_Kinematics (No Gyro)/2(y_dot) -> y_dot/1, Integrator3/1
  Qbot2_Diff_Drive_Kinematics/1(vC) -> Qbot2_Kinematics (No Gyro)/1(vC), vC/1
  vL/1 -> Qbot2_Diff_Drive_Kinematics/1(vL)
  vR/1 -> Qbot2_Diff_Drive_Kinematics/2(vR)
  Integrator2/1 -> x/1
  Integrator3/1 -> y/1
  Qbot2_Diff_Drive_Kinematics/2(Omega) -> Qbot2_Kinematics (No Gyro)/2(Omega), Omega/1

== system Obs_Avoi_with_sta_lin/QBot 2e Inverse Kinematics (Forward Velocity and Angular Velocity into Left and Right Wheel Velocity) ==
  vC : Inport
  Omega : Inport  Port=2
  Qbot2_Inverse_Kinematics (Forward Velocity and Angular Velocity into Left and Right Wheel Vellocity) : MATLAB Function  TreatAsAtomicUnit=on
  vR : Outport  VectorParamsAs1DForOutWhenUnconnected=off
  vL : Outport  Port=2  VectorParamsAs1DForOutWhenUnconnected=off
  wires:
  vC/1 -> Qbot2_Inverse_Kinematics (Forward Velocity and Angular Velocity into Left and Right Wheel Vellocity)/1(vC)
  Qbot2_Inverse_Kinematics (Forward Velocity and Angular Velocity into Left and Right Wheel Vellocity)/1(vR) -> vR/1
  Omega/1 -> Qbot2_Inverse_Kinematics (Forward Velocity and Angular Velocity into Left and Right Wheel Vellocity)/2(Omega)
  Qbot2_Inverse_Kinematics (Forward Velocity and Angular Velocity into Left and Right Wheel Vellocity)/2(vL) -> vL/1

== system Obs_Avoi_with_sta_lin/Video Compressed Display (Depth) ==
  In1 : Inport
  Channel : quarc_library/Signal Routing/Channel  channel=0  buffer_size=1
  Image Compress : quarc_library/Image Processing/Generic/Image Compress  algorithm=JPEG  source=Internal dialog parameter  quality=quality  output_dim=-1
  Video Display : quarc_library/Multimedia/Video Display  Tag=|  sample_time=sample_time  use_hardware=on
      | Obs_Avoi_with_sta_lin/Video Compressed
      | Display (Depth)/Video Display
  wires:
  Channel/1 -> Video Display/1
  In1/1 -> Image Compress/1
  Image Compress/1 -> Channel/1

== system Obs_Avoi_with_sta_lin/Video Compressed Display (RGB) ==
  In1 : Inport
  Channel : quarc_library/Signal Routing/Channel  channel=1  buffer_size=1
  Image Compress : quarc_library/Image Processing/Generic/Image Compress  algorithm=JPEG  source=Internal dialog parameter  quality=quality  output_dim=-1
  Video Display : quarc_library/Multimedia/Video Display  Tag=|  sample_time=sample_time  use_hardware=on
      | Obs_Avoi_with_sta_lin/Video Compressed
      | Display (RGB)/Video Display
  wires:
  Image Compress/1 -> Channel/1
  In1/1 -> Image Compress/1
  Channel/1 -> Video Display/1

== system Obs_Avoi_with_sta_lin/Video Compressed Display (RGB)  ==
  In1 : Inport
  Channel : quarc_library/Signal Routing/Channel  channel=0  buffer_size=1
  Image Compress : quarc_library/Image Processing/Generic/Image Compress  algorithm=JPEG  source=Internal dialog parameter  quality=quality  output_dim=-1
  Video Display : quarc_library/Multimedia/Video Display  Tag=|  sample_time=sample_time  use_hardware=on
      | Obs_Avoi_with_sta_lin/Video Compressed
      | Display (RGB) /Video Display
  wires:
  Channel/1 -> Video Display/1
  In1/1 -> Image Compress/1
  Image Compress/1 -> Channel/1

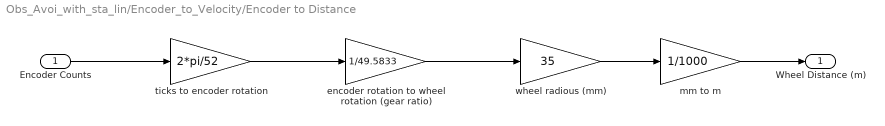
== system Obs_Avoi_with_sta_lin/Encoder_to_Velocity/Encoder to Distance ==
  Encoder Counts : Inport
  " encoder rotation to wheel rotation (gear ratio)" : Gain  Gain=1/49.5833
  mm to m : Gain  Gain=1/1000
  ticks to encoder rotation : Gain  Gain=2*pi/52
  wheel radious (mm) : Gain  Gain=35
  Wheel Distance (m) : Outport  VectorParamsAs1DForOutWhenUnconnected=off
  wires:
  Encoder Counts/1 -> ticks to encoder rotation/1
  ticks to encoder rotation/1 -> " encoder rotation to wheel rotation (gear ratio)"/1
  " encoder rotation to wheel rotation (gear ratio)"/1 -> wheel radious (mm)/1
  wheel radious (mm)/1 -> mm to m/1
  mm to m/1 -> Wheel Distance (m)/1

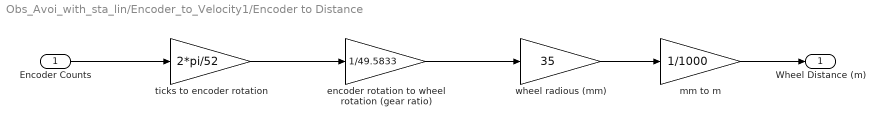
== system Obs_Avoi_with_sta_lin/Encoder_to_Velocity1/Encoder to Distance ==
  Encoder Counts : Inport
  " encoder rotation to wheel rotation (gear ratio)" : Gain  Gain=1/49.5833
  mm to m : Gain  Gain=1/1000
  ticks to encoder rotation : Gain  Gain=2*pi/52
  wheel radious (mm) : Gain  Gain=35
  Wheel Distance (m) : Outport  VectorParamsAs1DForOutWhenUnconnected=off
  wires:
  mm to m/1 -> Wheel Distance (m)/1
  wheel radious (mm)/1 -> mm to m/1
  " encoder rotation to wheel rotation (gear ratio)"/1 -> wheel radious (mm)/1
  ticks to encoder rotation/1 -> " encoder rotation to wheel rotation (gear ratio)"/1
  Encoder Counts/1 -> ticks to encoder rotation/1

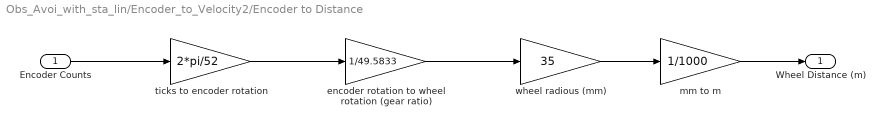
== system Obs_Avoi_with_sta_lin/Encoder_to_Velocity2/Encoder to Distance ==
  Encoder Counts : Inport
  " encoder rotation to wheel rotation (gear ratio)" : Gain  Gain=1/49.5833
  mm to m : Gain  Gain=1/1000
  ticks to encoder rotation : Gain  Gain=2*pi/52
  wheel radious (mm) : Gain  Gain=35
  Wheel Distance (m) : Outport  VectorParamsAs1DForOutWhenUnconnected=off
  wires:
  Encoder Counts/1 -> ticks to encoder rotation/1
  ticks to encoder rotation/1 -> " encoder rotation to wheel rotation (gear ratio)"/1
  " encoder rotation to wheel rotation (gear ratio)"/1 -> wheel radious (mm)/1
  wheel radious (mm)/1 -> mm to m/1
  mm to m/1 -> Wheel Distance (m)/1

== system Obs_Avoi_with_sta_lin/Encoder_to_Velocity3/Encoder to Distance ==
  Encoder Counts : Inport
  " encoder rotation to wheel rotation (gear ratio)" : Gain  Gain=1/49.5833
  mm to m : Gain  Gain=1/1000
  ticks to encoder rotation : Gain  Gain=2*pi/52
  wheel radious (mm) : Gain  Gain=35
  Wheel Distance (m) : Outport  VectorParamsAs1DForOutWhenUnconnected=off
  wires:
  mm to m/1 -> Wheel Distance (m)/1
  wheel radious (mm)/1 -> mm to m/1
  " encoder rotation to wheel rotation (gear ratio)"/1 -> wheel radious (mm)/1
  ticks to encoder rotation/1 -> " encoder rotation to wheel rotation (gear ratio)"/1
  Encoder Counts/1 -> ticks to encoder rotation/1

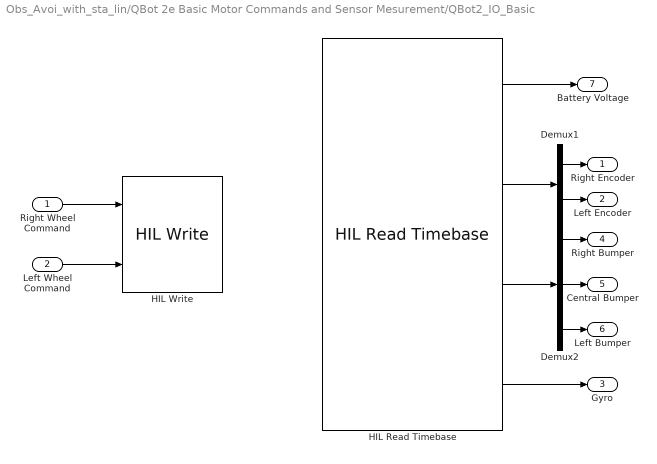
== system Obs_Avoi_with_sta_lin/QBot 2e Basic Motor Commands and Sensor Mesurement/QBot2_IO_Basic ==
  Right Wheel Command : Inport
  Left Wheel Command : Inport  Port=2
  Demux1 : Demux  Outputs=2
  Demux2 : Demux  Outputs=3
  HIL Read Timebase : quarc_library/Data Acquisition/Generic/Timebases/HIL Read Timebase  object_name=HIL-1  clock=0  analog_channels=0  encoder_channels=0:1  digital_channels=28:30  other_channels=1002  active=on  vector_output=on  data_type_mode=Inherit via back propagation  encoder_data_type=double  digital_data_type=boolean  overflow_mode=Synchronize (for simulated cards only)  samples_in_buffer=1+0*max(ceil(1/qc_get_step_size), 1)
  HIL Write : quarc_library/Data Acquisition/Generic/Immediate I//O/HIL Write  object_name=HIL-1  analog_channels=[]  pwm_channels=[]  digital_channels=[]  other_channels=[2000:2001]  sample_time=-1  active=on  vector_input=off
  Right Encoder : Outport  VectorParamsAs1DForOutWhenUnconnected=off
  Left Encoder : Outport  Port=2  VectorParamsAs1DForOutWhenUnconnected=off
  Gyro : Outport  Port=3  VectorParamsAs1DForOutWhenUnconnected=off
  Right Bumper : Outport  Port=4  VectorParamsAs1DForOutWhenUnconnected=off
  Central Bumper : Outport  Port=5  VectorParamsAs1DForOutWhenUnconnected=off
  Left Bumper : Outport  Port=6  VectorParamsAs1DForOutWhenUnconnected=off
  Battery Voltage : Outport  Port=7  VectorParamsAs1DForOutWhenUnconnected=off
  wires:
  HIL Read Timebase/1 -> Battery Voltage/1
  HIL Read Timebase/3 -> Demux2/1
  HIL Read Timebase/4 -> Gyro/1
  Demux1/1 -> Right Encoder/1
  Demux1/2 -> Left Encoder/1
  Right Wheel Command/1 -> HIL Write/1
  Left Wheel Command/1 -> HIL Write/2
  HIL Read Timebase/2 -> Demux1/1
  Demux2/1 -> Right Bumper/1
  Demux2/2 -> Central Bumper/1
  Demux2/3 -> Left Bumper/1

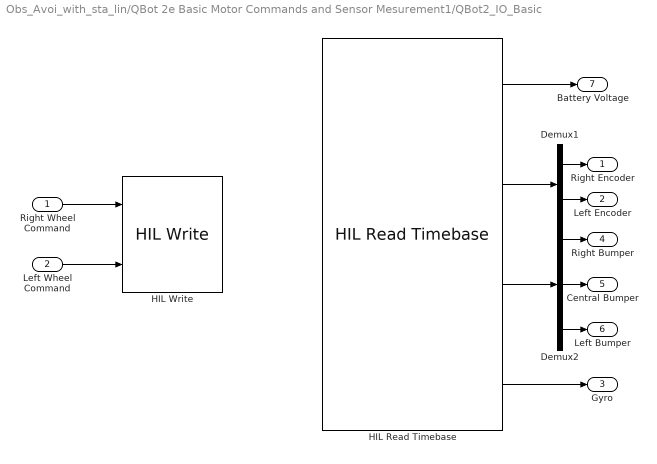
== system Obs_Avoi_with_sta_lin/QBot 2e Basic Motor Commands and Sensor Mesurement1/QBot2_IO_Basic ==
  Right Wheel Command : Inport
  Left Wheel Command : Inport  Port=2
  Demux1 : Demux  Outputs=2
  Demux2 : Demux  Outputs=3
  HIL Read Timebase : quarc_library/Data Acquisition/Generic/Timebases/HIL Read Timebase  object_name=HIL-1  clock=0  analog_channels=0  encoder_channels=0:1  digital_channels=28:30  other_channels=1002  active=on  vector_output=on  data_type_mode=Inherit via back propagation  encoder_data_type=double  digital_data_type=boolean  overflow_mode=Synchronize (for simulated cards only)  samples_in_buffer=1+0*max(ceil(1/qc_get_step_size), 1)
  HIL Write : quarc_library/Data Acquisition/Generic/Immediate I//O/HIL Write  object_name=HIL-1  analog_channels=[]  pwm_channels=[]  digital_channels=[]  other_channels=[2000:2001]  sample_time=-1  active=on  vector_input=off
  Right Encoder : Outport  VectorParamsAs1DForOutWhenUnconnected=off
  Left Encoder : Outport  Port=2  VectorParamsAs1DForOutWhenUnconnected=off
  Gyro : Outport  Port=3  VectorParamsAs1DForOutWhenUnconnected=off
  Right Bumper : Outport  Port=4  VectorParamsAs1DForOutWhenUnconnected=off
  Central Bumper : Outport  Port=5  VectorParamsAs1DForOutWhenUnconnected=off
  Left Bumper : Outport  Port=6  VectorParamsAs1DForOutWhenUnconnected=off
  Battery Voltage : Outport  Port=7  VectorParamsAs1DForOutWhenUnconnected=off
  wires:
  HIL Read Timebase/1 -> Battery Voltage/1
  HIL Read Timebase/3 -> Demux2/1
  HIL Read Timebase/4 -> Gyro/1
  Demux1/1 -> Right Encoder/1
  Demux1/2 -> Left Encoder/1
  Right Wheel Command/1 -> HIL Write/1
  Left Wheel Command/1 -> HIL Write/2
  HIL Read Timebase/2 -> Demux1/1
  Demux2/1 -> Right Bumper/1
  Demux2/2 -> Central Bumper/1
  Demux2/3 -> Left Bumper/1

== system Obs_Avoi_with_sta_lin/QBot 2e Full Kinematics/Qbot2_Diff_Drive_Kinematics ==
  vL : Inport
  vR : Inport  Port=2
  Qbot2_Diff_Drive_Kinematics : MATLAB Function  TreatAsAtomicUnit=on
  vC : Outport  VectorParamsAs1DForOutWhenUnconnected=off
  Omega : Outport  Port=2  VectorParamsAs1DForOutWhenUnconnected=off
  wires:
  vL/1 -> Qbot2_Diff_Drive_Kinematics/1(vL)
  Qbot2_Diff_Drive_Kinematics/1(vC) -> vC/1
  vR/1 -> Qbot2_Diff_Drive_Kinematics/2(vR)
  Qbot2_Diff_Drive_Kinematics/2(Omega) -> Omega/1

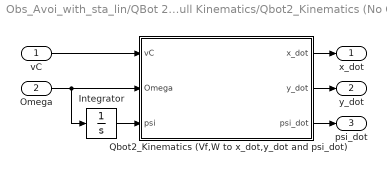
== system Obs_Avoi_with_sta_lin/QBot 2e Full Kinematics/Qbot2_Kinematics (No Gyro) ==
  vC : Inport
  Omega : Inport  Port=2
  Integrator : Integrator
  Qbot2_Kinematics (Vf,W to x_dot,y_dot and psi_dot) : MATLAB Function  TreatAsAtomicUnit=on
  x_dot : Outport  VectorParamsAs1DForOutWhenUnconnected=off
  y_dot : Outport  Port=2  VectorParamsAs1DForOutWhenUnconnected=off
  psi_dot : Outport  Port=3  VectorParamsAs1DForOutWhenUnconnected=off
  wires:
  Qbot2_Kinematics (Vf,W to x_dot,y_dot and psi_dot)/3(psi_dot) -> psi_dot/1
  Integrator/1 -> Qbot2_Kinematics (Vf,W to x_dot,y_dot and psi_dot)/3(psi)
  vC/1 -> Qbot2_Kinematics (Vf,W to x_dot,y_dot and psi_dot)/1(vC)
  Qbot2_Kinematics (Vf,W to x_dot,y_dot and psi_dot)/1(x_dot) -> x_dot/1
  Omega/1 -> Integrator/1, Qbot2_Kinematics (Vf,W to x_dot,y_dot and psi_dot)/2(Omega)
  Qbot2_Kinematics (Vf,W to x_dot,y_dot and psi_dot)/2(y_dot) -> y_dot/1

== system Obs_Avoi_with_sta_lin/QBot 2e Full Kinematics1/Qbot2_Diff_Drive_Kinematics ==
  vL : Inport
  vR : Inport  Port=2
  Qbot2_Diff_Drive_Kinematics : MATLAB Function  TreatAsAtomicUnit=on
  vC : Outport  VectorParamsAs1DForOutWhenUnconnected=off
  Omega : Outport  Port=2  VectorParamsAs1DForOutWhenUnconnected=off
  wires:
  vL/1 -> Qbot2_Diff_Drive_Kinematics/1(vL)
  Qbot2_Diff_Drive_Kinematics/1(vC) -> vC/1
  vR/1 -> Qbot2_Diff_Drive_Kinematics/2(vR)
  Qbot2_Diff_Drive_Kinematics/2(Omega) -> Omega/1
